simulink model "Charge_2_V1"  (R2017b)
settings: Solver=FixedStepDiscrete  StartTime=0.0  StopTime=1  FixedStep=0.001  RelTol=1e-3
PreLoadFcn:
  | librarySetup
  | eval([bdroot,'_startup']) %Calling [modelName]_startup.m
undefined symbols (not defined in the file or in its folder): A0, A1, Car1__Authorize, Car2_Authorize, CON2, CON3, CON4, Control_Mode_In, CurrentSP, D10, D12, D13, D2, D3, D4, D5, D6, D7, D8, Frequency_High_Point, Frequency_Low_Point, Frequency_Mid_high, Frequency_Mid_low, HVol_High_Point, HVol_Low_Point, HVol_Mid_high, HVol_Mid_low, HVoltage_Factor, SeconCar_ThreePhase, V_Current_five, V_Current_four, V_Current_one, V_Current_six, V_Current_three, V_Current_two, V_Frequency, V_MaxPliot, V_MinPliot, Vol_High_Point, Vol_Low_Point, Vol_Mid_high, Vol_Mid_low, Voltage_Factor, Voltage_Mode_Test
libraries: simulink x331, HANcoder_STM32_Target x30, powerlib_meascontrol x8, simulink_extras x2
(part 13 of 13)

== system Charge_2_V1/HANcoder STM32 Target - E407-STM32 algorithm/Energy Meter1/Energy_Meter_Recieve/Subsystem1/f1/Current_Phase1/Read_Gyro2/UART send ==
  In1 : Inport
  Level-2 M-file S-Function : M-S-Function  FunctionName=sfcn_uart_send  Parameters=tsamp
  Term1 : Terminator
  wires:
  Level-2 M-file S-Function/1 -> Term1/1
  In1/1 -> Level-2 M-file S-Function/1

== system Charge_2_V1/HANcoder STM32 Target - E407-STM32 algorithm/Energy Meter1/Energy_Meter_Recieve/Subsystem1/f1/Current_Phase1/Read_Gyro3/UART send ==
  In1 : Inport
  Level-2 M-file S-Function : M-S-Function  FunctionName=sfcn_uart_send  Parameters=tsamp
  Term1 : Terminator
  wires:
  Level-2 M-file S-Function/1 -> Term1/1
  In1/1 -> Level-2 M-file S-Function/1

== system Charge_2_V1/HANcoder STM32 Target - E407-STM32 algorithm/Energy Meter1/Energy_Meter_Recieve/Subsystem1/f1/Current_Phase1/Read_Gyro4/UART send ==
  In1 : Inport
  Level-2 M-file S-Function : M-S-Function  FunctionName=sfcn_uart_send  Parameters=tsamp
  Term1 : Terminator
  wires:
  Level-2 M-file S-Function/1 -> Term1/1
  In1/1 -> Level-2 M-file S-Function/1

== system Charge_2_V1/HANcoder STM32 Target - E407-STM32 algorithm/Energy Meter1/Energy_Meter_Recieve/Subsystem1/f1/Current_phase2/Read_Gyro5/UART send ==
  In1 : Inport
  Level-2 M-file S-Function : M-S-Function  FunctionName=sfcn_uart_send  Parameters=tsamp
  Term1 : Terminator
  wires:
  In1/1 -> Level-2 M-file S-Function/1
  Level-2 M-file S-Function/1 -> Term1/1

== system Charge_2_V1/HANcoder STM32 Target - E407-STM32 algorithm/Energy Meter1/Energy_Meter_Recieve/Subsystem1/f1/Current_phase2/Read_Gyro7/UART send ==
  In1 : Inport
  Level-2 M-file S-Function : M-S-Function  FunctionName=sfcn_uart_send  Parameters=tsamp
  Term1 : Terminator
  wires:
  Level-2 M-file S-Function/1 -> Term1/1
  In1/1 -> Level-2 M-file S-Function/1

== system Charge_2_V1/HANcoder STM32 Target - E407-STM32 algorithm/Energy Meter1/Energy_Meter_Recieve/Subsystem1/f1/Current_phase2/Read_Gyro8/UART send ==
  In1 : Inport
  Level-2 M-file S-Function : M-S-Function  FunctionName=sfcn_uart_send  Parameters=tsamp
  Term1 : Terminator
  wires:
  In1/1 -> Level-2 M-file S-Function/1
  Level-2 M-file S-Function/1 -> Term1/1

== system Charge_2_V1/HANcoder STM32 Target - E407-STM32 algorithm/Energy Meter1/Energy_Meter_Recieve/Subsystem1/f1/Current_phase2/Read_Gyro9/UART send ==
  In1 : Inport
  Level-2 M-file S-Function : M-S-Function  FunctionName=sfcn_uart_send  Parameters=tsamp
  Term1 : Terminator
  wires:
  Level-2 M-file S-Function/1 -> Term1/1
  In1/1 -> Level-2 M-file S-Function/1

== system Charge_2_V1/HANcoder STM32 Target - E407-STM32 algorithm/Energy Meter1/Energy_Meter_Recieve/Subsystem1/f1/Subsystem/Read_Gyro10/UART send ==
  In1 : Inport
  Level-2 M-file S-Function : M-S-Function  FunctionName=sfcn_uart_send  Parameters=tsamp
  Term1 : Terminator
  wires:
  Level-2 M-file S-Function/1 -> Term1/1
  In1/1 -> Level-2 M-file S-Function/1

== system Charge_2_V1/HANcoder STM32 Target - E407-STM32 algorithm/Energy Meter1/Energy_Meter_Recieve/Subsystem1/f1/Subsystem/Read_Gyro12/UART send ==
  In1 : Inport
  Level-2 M-file S-Function : M-S-Function  FunctionName=sfcn_uart_send  Parameters=tsamp
  Term1 : Terminator
  wires:
  In1/1 -> Level-2 M-file S-Function/1
  Level-2 M-file S-Function/1 -> Term1/1

== system Charge_2_V1/HANcoder STM32 Target - E407-STM32 algorithm/Energy Meter1/Energy_Meter_Recieve/Subsystem1/f1/Subsystem/Read_Gyro13/UART send ==
  In1 : Inport
  Level-2 M-file S-Function : M-S-Function  FunctionName=sfcn_uart_send  Parameters=tsamp
  Term1 : Terminator
  wires:
  Level-2 M-file S-Function/1 -> Term1/1
  In1/1 -> Level-2 M-file S-Function/1

== system Charge_2_V1/HANcoder STM32 Target - E407-STM32 algorithm/Energy Meter1/Energy_Meter_Recieve/Subsystem1/f1/Subsystem/Read_Gyro14/UART send ==
  In1 : Inport
  Level-2 M-file S-Function : M-S-Function  FunctionName=sfcn_uart_send  Parameters=tsamp
  Term1 : Terminator
  wires:
  In1/1 -> Level-2 M-file S-Function/1
  Level-2 M-file S-Function/1 -> Term1/1

== system Charge_2_V1/HANcoder STM32 Target - E407-STM32 algorithm/Energy Meter1/Energy_Meter_Recieve/Subsystem1/f2/Current_Phase1/Read_Gyro1/UART send ==
  In1 : Inport
  Level-2 M-file S-Function : M-S-Function  FunctionName=sfcn_uart_send  Parameters=tsamp
  Term1 : Terminator
  wires:
  In1/1 -> Level-2 M-file S-Function/1
  Level-2 M-file S-Function/1 -> Term1/1

== system Charge_2_V1/HANcoder STM32 Target - E407-STM32 algorithm/Energy Meter1/Energy_Meter_Recieve/Subsystem1/f2/Current_Phase1/Read_Gyro2/UART send ==
  In1 : Inport
  Level-2 M-file S-Function : M-S-Function  FunctionName=sfcn_uart_send  Parameters=tsamp
  Term1 : Terminator
  wires:
  In1/1 -> Level-2 M-file S-Function/1
  Level-2 M-file S-Function/1 -> Term1/1

== system Charge_2_V1/HANcoder STM32 Target - E407-STM32 algorithm/Energy Meter1/Energy_Meter_Recieve/Subsystem1/f2/Current_Phase1/Read_Gyro3/UART send ==
  In1 : Inport
  Level-2 M-file S-Function : M-S-Function  FunctionName=sfcn_uart_send  Parameters=tsamp
  Term1 : Terminator
  wires:
  In1/1 -> Level-2 M-file S-Function/1
  Level-2 M-file S-Function/1 -> Term1/1

== system Charge_2_V1/HANcoder STM32 Target - E407-STM32 algorithm/Energy Meter1/Energy_Meter_Recieve/Subsystem1/f2/Current_Phase1/Read_Gyro4/UART send ==
  In1 : Inport
  Level-2 M-file S-Function : M-S-Function  FunctionName=sfcn_uart_send  Parameters=tsamp
  Term1 : Terminator
  wires:
  In1/1 -> Level-2 M-file S-Function/1
  Level-2 M-file S-Function/1 -> Term1/1

== stateflow chart Charge_2_V1/HANcoder STM32 Target - E407-STM32 algorithm/Car2/Chart1 ==
  settings: updateMethod=DISCRETE  sampleTime=2
  state Idle
    Switch=0;
    Pwm=1;
    State=1;
  state StateA
    Switch=0;
    Pwm=1;
    State=2;
  state StateF
    Switch=0;
    Pwm=1;
    State=7;
  state StateB
    Switch=0;
    Pwm=0.55;
    State=3;
  state StateE
    Switch=0;
    Pwm=1;
    State=6;
  state StateCD
    Switch=1;
    Pwm=inPWM;
    State=4;
  state StateB1
    Switch=1;
    Pwm=1;
    State=4;
  state StateE1
    Switch=1;
    Pwm=inPWM;
    State=4;
  (default) -> Idle
  StateF -> Idle : [!Maxvalue<-10.5]
  Idle -> StateA : [Maxvalue>10.5 && Maxvalue<15]
  StateA -> Idle [order 2] : [Maxvalue>15]
  StateB -> StateA [order 2] : [Maxvalue>10.5 ]
  StateA -> StateB [order 1] : [Maxvalue>7.5 && Maxvalue<10.5 ]
  StateE -> StateA : [!Maxvalue<1.5 ]
  StateCD -> StateF [order 2] : [Maxvalue<-10.5]
  StateB1 -> StateB : [after(2,sec)]
  StateE1 -> StateE [order 1] : [after(2,sec) && (Maxvalue<1.5 || Minvalue>-9.5) ]
  StateCD -> StateB [order 1] : [(Maxvalue>7.5 && Minvalue<-9.5) ]
  StateB -> StateCD [order 1] : [Maxvalue>1.5 && Maxvalue<7.5 && Minvalue<-9.5 && Start>0 ]
  StateCD -> StateE1 [order 3] : [Maxvalue<1.5 || Minvalue>-9.5]
  StateCD -> StateB1 [order 5] : [ Start<1]
  StateE1 -> StateCD [order 2] : [after(2,sec) && (Maxvalue>1.5 || Minvalue<-9.5) ]
  StateCD -> StateCD [order 4] : [Maxvalue>1.5 && Maxvalue<7.5 && Minvalue<-9.5 && Start>0]
  data: Switch output boolean; Maxvalue input single; Minvalue input single; Pwm output single; inPWM input single; State output int8; Start input boolean

== stateflow chart Charge_2_V1/HANcoder STM32 Target - E407-STM32 algorithm/Car1/Chart1 ==
  settings: updateMethod=DISCRETE  sampleTime=2
  state Idle
    Switch=0;
    Pwm=1;
    State=1;
  state StateA
    Switch=0;
    Pwm=1;
    State=2;
  state StateF
    Switch=0;
    Pwm=1;
    State=7;
  state StateB
    Switch=0;
    Pwm=0.55;
    State=3;
  state StateE
    Switch=0;
    Pwm=1;
    State=6;
  state StateCD
    Switch=1;
    Pwm=inPWM;
    State=4;
  state StateB1
    Switch=1;
    Pwm=1;
    State=4;
  state StateE1
    Switch=1;
    Pwm=inPWM;
    State=4;
  (default) -> Idle
  StateF -> Idle : [!Maxvalue<-10.5]
  Idle -> StateA : [Maxvalue>10.5 && Maxvalue<15]
  StateA -> Idle [order 2] : [Maxvalue>15]
  StateB -> StateA [order 2] : [Maxvalue>10.5 ]
  StateA -> StateB [order 1] : [Maxvalue>7.5 && Maxvalue<10.5 ]
  StateE -> StateA : [!Maxvalue<1.5 ]
  StateCD -> StateF [order 2] : [Maxvalue<-10.5]
  StateB1 -> StateB : [after(2,sec)]
  StateE1 -> StateE [order 1] : [after(2,sec) && (Maxvalue<1.5 || Minvalue>-9.5) ]
  StateCD -> StateB [order 1] : [(Maxvalue>7.5 && Minvalue<-9.5) ]
  StateB -> StateCD [order 1] : [Maxvalue>1.5 && Maxvalue<7.5 && Minvalue<-9.5 && Start>0 ]
  StateCD -> StateE1 [order 3] : [Maxvalue<1.5 || Minvalue>-9.5]
  StateCD -> StateB1 [order 5] : [ Start<1]
  StateE1 -> StateCD [order 2] : [after(2,sec) && (Maxvalue>1.5 || Minvalue<-9.5) ]
  StateCD -> StateCD [order 4] : [Maxvalue>1.5 && Maxvalue<7.5 && Minvalue<-9.5 && Start>0]
  data: Switch output boolean; Maxvalue input single; Minvalue input single; Pwm output single; inPWM input single; State output int8; Start input boolean

== stateflow chart Charge_2_V1/HANcoder STM32 Target - E407-STM32 algorithm/Current_SP/Current_Limit1/Chart1 ==
  settings: updateMethod=DISCRETE
  state Idle
    Limit_Out=Limit_In;
    State=1;
  state StateA
    Limit_Out=16;
    State=2;
  state StateB
    Limit_Out=Limit_In;
    State=3;
  (default) -> Idle
  Idle -> StateA : [SecondCarOn>0]
  StateB -> Idle [order 1] : [SecondCarOn<1]
  StateA -> StateB : [after(60,sec)]
  StateB -> StateB [order 2] : [SecondCarOn>0]
  data: State output int8; Limit_In input; SecondCarOn input; Limit_Out output
